simulink model "untitled"  (R2016a)
settings: Solver=VariableStepAuto  StartTime=0.0  StopTime=10.0  RelTol=1e-3
libraries: simrfV2elements x6, simrfV2util1 x5, fl_lib x4, simrfV2sources1 x1
settings Model: Creator=syf  LastModifiedBy=syf

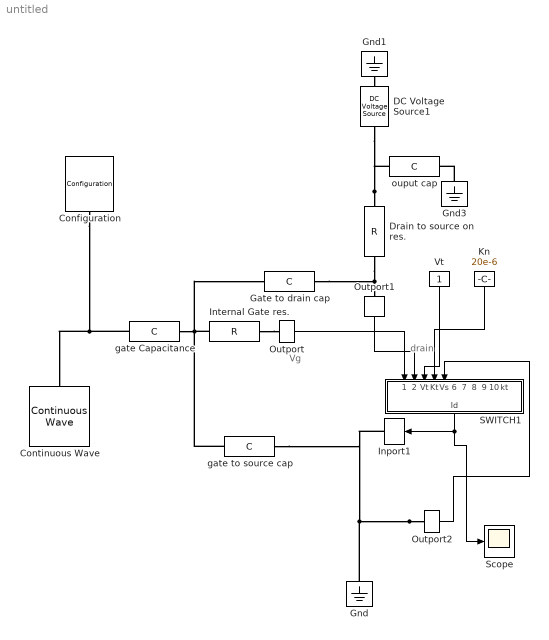
== system untitled ==
  note: drain
  note: Vg
  Configuration : simrfV2util1/Configuration  AutoFreq=on  Tones=[] Hz  Harmonics=[]  NormalizeCarrierPower=on  SolverType=Auto  StepSize=1e-6 s  AddNoise=on  Temperature=290.0 K  SolverDelFlag=0
  Continuous Wave : simrfV2sources1/Continuous Wave  CWSourceType=Ideal voltage  Z0=0  IVoltage=5 V  ICurrent=0 A  MagPower=0 W  QVoltage=0 V  QCurrent=0 A  AnglePower=0  CarrierFreq=0 Hz  InternalGrounding=on
  DC Voltage Source1 : fl_lib/Electrical/Electrical Sources/DC Voltage Source  v0=5 V
  Drain to source on res. : simrfV2elements/R  classname=resistor  Resistance=0.005 Ohm  AddNoise=on
  "Gate to drain cap " : simrfV2elements/C  classname=capacitor  Capacitance=0.3e-9 F
  Gnd : fl_lib/Electrical/Electrical Elements/Electrical Reference
  Gnd1 : fl_lib/Electrical/Electrical Elements/Electrical Reference
  Gnd3 : fl_lib/Electrical/Electrical Elements/Electrical Reference
  Inport1 : simrfV2util1/Inport  SimulinkInputSignalType=Ideal voltage  CarrierFreq=0 Hz  ZS=0  InternalGrounding=on
  Internal Gate res. : simrfV2elements/R  classname=resistor  Resistance=1.5 Ohm  AddNoise=on
  Kn : Constant  Value=20e-6
  Outport : simrfV2util1/Outport  SensorType=Ideal voltage  OutputFormat=Complex Baseband  CarrierFreq=0 Hz  ZL=Inf  InternalGrounding=on  StepSize=1e-6 s  AutoStep=on
  Outport1 : simrfV2util1/Outport  SensorType=Ideal voltage  OutputFormat=Complex Baseband  CarrierFreq=0 Hz  ZL=Inf  InternalGrounding=on  StepSize=1e-6 s  AutoStep=on
  Outport2 : simrfV2util1/Outport  SensorType=Ideal voltage  OutputFormat=Complex Baseband  CarrierFreq=0 Hz  ZL=Inf  InternalGrounding=on  StepSize=1e-6 s  AutoStep=on
  SWITCH1 : Subsystem
  Scope : Scope
  Vt : Constant
  gate Capacitance : simrfV2elements/C  classname=capacitor  Capacitance=0.9667e-9 F
  gate to source cap : simrfV2elements/C  classname=capacitor  Capacitance=0.3667e-9 F
  "ouput cap " : simrfV2elements/C  classname=capacitor  Capacitance=65e-12 F
  wires:
  Outport/1 -> SWITCH1/1(Vg)
  Outport1/1 -> SWITCH1/2(Vd)
  SWITCH1/1(Id) -> Scope/1, Inport1/1
  Outport2/1 -> SWITCH1/5(Vs)
  Vt/1 -> SWITCH1/3(Vt)
  Kn/1 -> SWITCH1/4(Kt)
  connections:
  gate to source cap/LConn1 -- "Gate to drain cap "/LConn1 -- gate Capacitance/RConn1 -- Internal Gate res./LConn1
  Outport1/LConn1 -- "Gate to drain cap "/RConn1 -- Drain to source on res./RConn1
  Outport2/LConn1 -- Gnd/LConn1 -- gate to source cap/RConn1 -- Inport1/RConn1
  Configuration/LConn1 -- gate Capacitance/LConn1 -- Continuous Wave/LConn1
  Drain to source on res./LConn1 -- DC Voltage Source1/LConn1 -- "ouput cap "/LConn1
  Internal Gate res./RConn1 -- Outport/LConn1
  Gnd1/LConn1 -- DC Voltage Source1/RConn1
  Gnd3/LConn1 -- "ouput cap "/RConn1

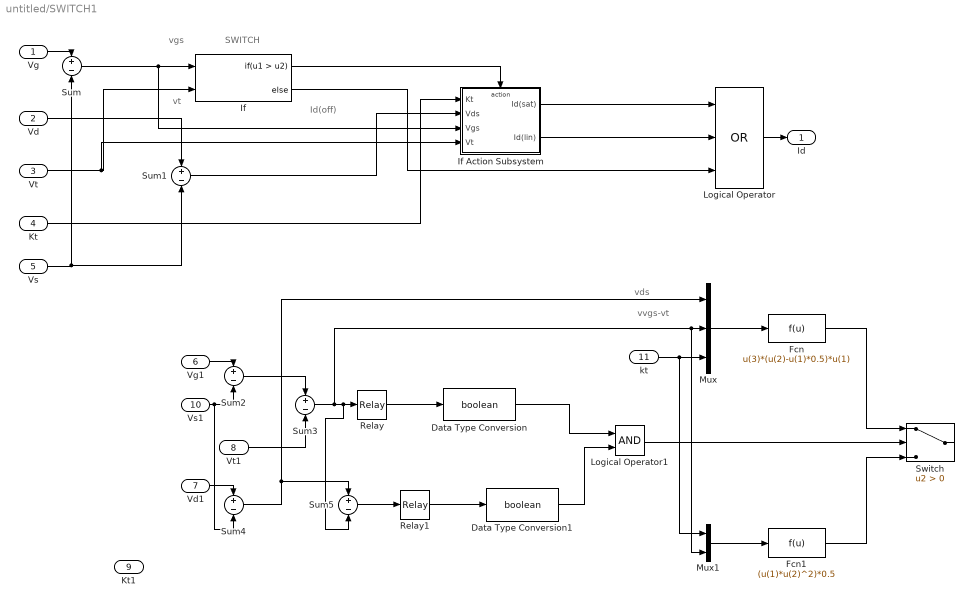
== system untitled/SWITCH1 ==
  note: vvgs-vt
  note: vds
  note: SWITCH
  note: Id(off)
  note: vt
  note: vgs
  Vg : Inport
  Vd : Inport  Port=2
  Vt : Inport  Port=3
  Kt : Inport  Port=4
  Vs : Inport  Port=5
  Vg1 : Inport  Port=6
  Vd1 : Inport  Port=7
  Vt1 : Inport  Port=8
  Kt1 : Inport  Port=9
  Vs1 : Inport  Port=10
  kt : Inport  Port=11
  Data Type Conversion : DataTypeConversion  OutDataTypeStr=boolean
  Data Type Conversion1 : DataTypeConversion  OutDataTypeStr=boolean
  Fcn : Fcn  Expr=u(3)*(u(2)-u(1)*0.5)*u(1)
  Fcn1 : Fcn  Expr=(u(1)*u(2)^2)*0.5
  If : If  NumInputs=2  IfExpression=u1 > u2
  If Action Subsystem : Subsystem  TreatAsAtomicUnit=on
  Logical Operator : Logic  Operator=OR  Inputs=3  AllPortsSameDT=off  OutDataTypeStr=boolean
  Logical Operator1 : Logic  AllPortsSameDT=off  OutDataTypeStr=boolean
  Mux : Mux  Inputs=3
  Mux1 : Mux  Inputs=2
  Relay : Relay
  Relay1 : Relay
  Sum{,1..5} (6 alike) : Sum  Inputs=+-
  Switch : Switch  Criteria=u2 > Threshold
  Id : Outport
  wires:
  Vt/1 -> If Action Subsystem/4(Vt), If/2
  If Action Subsystem/2(Id(lin)) -> Logical Operator/2
  Kt/1 -> If Action Subsystem/1(Kt)
  If/1 -> If Action Subsystem/Action
  If/2 -> Logical Operator/3
  If Action Subsystem/1(Id(sat)) -> Logical Operator/1
  Vg/1 -> Sum/1
  Vs/1 -> Sum1/2, Sum/2
  Sum/1 -> If Action Subsystem/3(Vgs), If/1
  Vd/1 -> Sum1/1
  Sum1/1 -> If Action Subsystem/2(Vds)
  Logical Operator/1 -> Id/1
  Relay/1 -> Data Type Conversion/1
  Vt1/1 -> Sum3/2
  Vg1/1 -> Sum2/1
  Vs1/1 -> Sum2/2, Sum4/2
  Sum2/1 -> Sum3/1
  Vd1/1 -> Sum4/1
  Relay1/1 -> Data Type Conversion1/1
  Sum5/1 -> Relay1/1
  Data Type Conversion/1 -> Logical Operator1/1
  Data Type Conversion1/1 -> Logical Operator1/2
  Logical Operator1/1 -> Switch/2
  Sum4/1 -> Mux/1, Sum5/1
  Mux/1 -> Fcn/1
  Fcn/1 -> Switch/1
  Sum3/1 -> Mux1/2, Mux/2, Sum5/2, Relay/1
  kt/1 -> Mux1/1, Mux/3
  Mux1/1 -> Fcn1/1
  Fcn1/1 -> Switch/3

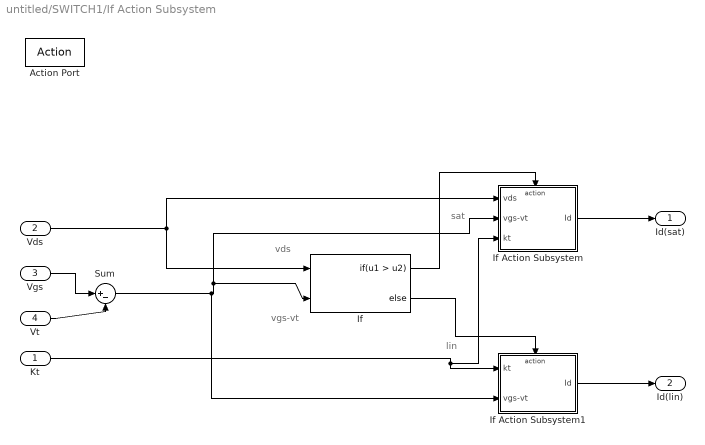
== system untitled/SWITCH1/If Action Subsystem ==
  note: lin
  note: sat
  note: vgs-vt
  note: vds
  Kt : Inport
  Vds : Inport  Port=2
  Vgs : Inport  Port=3
  Vt : Inport  Port=4
  Action Port : ActionPort
  If : If  NumInputs=2  IfExpression=u1 > u2
  If Action Subsystem : Subsystem  TreatAsAtomicUnit=on
  If Action Subsystem1 : Subsystem  TreatAsAtomicUnit=on
  Sum : Sum  Inputs=|+-
  Id(sat) : Outport
  Id(lin) : Outport  Port=2
  wires:
  Vds/1 -> If Action Subsystem/1(vds), If/1
  Kt/1 -> If Action Subsystem1/1(kt), If Action Subsystem/3(kt)
  If/2 -> If Action Subsystem1/Action
  If Action Subsystem/1(Id) -> Id(sat)/1
  Sum/1 -> If Action Subsystem1/2(vgs-vt), If Action Subsystem/2(vgs-vt), If/2
  Vt/1 -> Sum/2
  Vgs/1 -> Sum/1
  If Action Subsystem1/1(Id) -> Id(lin)/1
  If/1 -> If Action Subsystem/Action

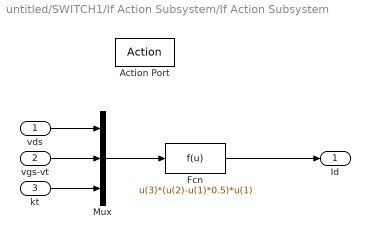
== system untitled/SWITCH1/If Action Subsystem/If Action Subsystem ==
  vds : Inport
  vgs-vt : Inport  Port=2
  kt : Inport  Port=3
  Action Port : ActionPort
  Fcn : Fcn  Expr=u(3)*(u(2)-u(1)*0.5)*u(1)
  Mux : Mux  Inputs=3
  Id : Outport
  wires:
  vds/1 -> Mux/1
  vgs-vt/1 -> Mux/2
  kt/1 -> Mux/3
  Mux/1 -> Fcn/1
  Fcn/1 -> Id/1

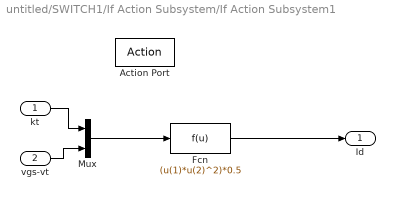
== system untitled/SWITCH1/If Action Subsystem/If Action Subsystem1 ==
  kt : Inport
  vgs-vt : Inport  Port=2
  Action Port : ActionPort
  Fcn : Fcn  Expr=(u(1)*u(2)^2)*0.5
  Mux : Mux  Inputs=2
  Id : Outport
  wires:
  vgs-vt/1 -> Mux/2
  kt/1 -> Mux/1
  Mux/1 -> Fcn/1
  Fcn/1 -> Id/1
